simulink model "Autopilot"  (Simulink 8.0)
settings: configuration reference "configSetObj_autopilot" (kept outside this file)
undefined symbols (not defined in the file or in its folder): dispGain, intGain, rateGain
settings Model: Creator=The MathWorks Inc.  LastModifiedBy=klindqvi  CovMetricSettings=dcmtrwe  CovHTMLOptions=-aTS=1 -bRG=1 -bTC=1 -hTR=0 -nFC=0 -scm=1 -bcm=1 -xEv=0  CovSaveSingleToWorkspaceVar=off  CovCumulativeReport=on  CovModelRefEnable=off  ExtModeTrigMode=oneshot  ExtModeArmWhenConnect=off  ExtModeAutoUpdateStatusClock=off
settings ConfigSet: SourceLocation=Base Workspace

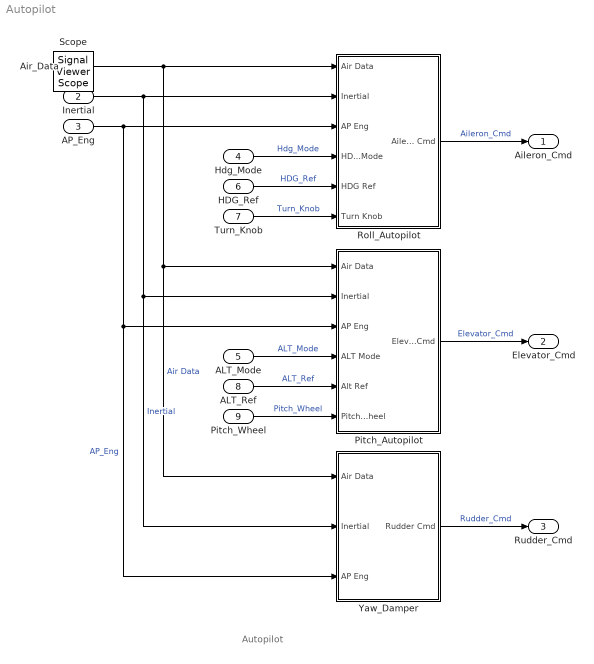
== system Autopilot ==
  note: Autopilot
  Air_Data : Inport  OutDataTypeStr=Bus: slBus_AirData  SampleTime=[0.025000000000000001,0]  BusOutputAsStruct=on
  Inertial : Inport  Port=2  OutDataTypeStr=Bus: slBus_Inertial  SampleTime=[0.025000000000000001,0]  BusOutputAsStruct=on
  AP_Eng : Inport  Port=3  OutDataTypeStr=boolean  PortDimensions=1  SampleTime=[0.025000000000000001,0]
  Hdg_Mode : Inport  Port=4  OutDataTypeStr=boolean  PortDimensions=1  SampleTime=[0.025000000000000001,0]
  ALT_Mode : Inport  Port=5  OutDataTypeStr=boolean  PortDimensions=1  SampleTime=[0.025000000000000001,0]
  HDG_Ref : Inport  Port=6  OutDataTypeStr=double  PortDimensions=1  SampleTime=[0.025000000000000001,0]
  Turn_Knob : Inport  Port=7  OutDataTypeStr=double  PortDimensions=1  SampleTime=[0.025000000000000001,0]
  ALT_Ref : Inport  Port=8  OutDataTypeStr=double  PortDimensions=1  SampleTime=[0.025000000000000001,0]
  Pitch_Wheel : Inport  Port=9  OutDataTypeStr=double  PortDimensions=1  SampleTime=[0.025000000000000001,0]
  Pitch_Autopilot : Subsystem  TreatAsAtomicUnit=on
  Roll_Autopilot : Subsystem  TreatAsAtomicUnit=on
  Yaw_Damper : Subsystem  TreatAsAtomicUnit=on
  Aileron_Cmd : Outport  OutDataTypeStr=double  PortDimensions=1  SampleTime=[0.025000000000000001,0]
  Elevator_Cmd : Outport  Port=2  OutDataTypeStr=double  PortDimensions=1  SampleTime=[0.025000000000000001,0]
  Rudder_Cmd : Outport  Port=3  OutDataTypeStr=double  PortDimensions=1  SampleTime=[0.025000000000000001,0]
  Scope : SignalViewerScope  IOType=viewer  RefreshTime=0.035000
  wires:
  AP_Eng/1 -> Yaw_Damper/3(AP Eng), Pitch_Autopilot/3(AP Eng), Roll_Autopilot/3(AP Eng)  "AP_Eng"
  Pitch_Wheel/1 -> Pitch_Autopilot/6(Pitch Wheel)  "Pitch_Wheel"
  ALT_Ref/1 -> Pitch_Autopilot/5(Alt Ref)  "ALT_Ref"
  ALT_Mode/1 -> Pitch_Autopilot/4(ALT Mode)  "ALT_Mode"
  Turn_Knob/1 -> Roll_Autopilot/6(Turn Knob)  "Turn_Knob"
  HDG_Ref/1 -> Roll_Autopilot/5(HDG Ref)  "HDG_Ref"
  Hdg_Mode/1 -> Roll_Autopilot/4(HDG Mode)  "Hdg_Mode"
  Inertial/1 -> Yaw_Damper/2(Inertial), Pitch_Autopilot/2(Inertial), Roll_Autopilot/2(Inertial)  "Inertial"
  Air_Data/1 -> Yaw_Damper/1(Air Data), Pitch_Autopilot/1(Air Data), Roll_Autopilot/1(Air Data)  "Air Data"
  Yaw_Damper/1(Rudder Cmd) -> Rudder_Cmd/1  "Rudder_Cmd"
  Pitch_Autopilot/1(Elevator_Cmd) -> Elevator_Cmd/1  "Elevator_Cmd"
  Roll_Autopilot/1(Aileron Cmd) -> Aileron_Cmd/1  "Aileron_Cmd"

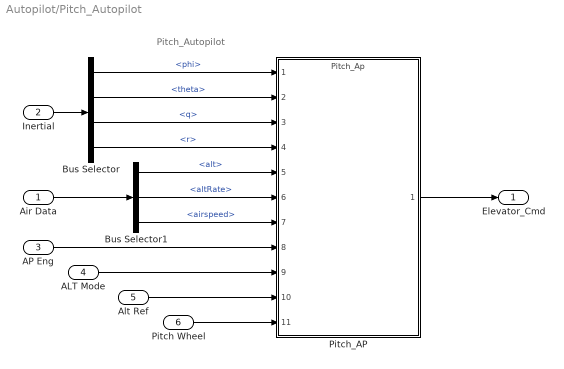
== system Autopilot/Pitch_Autopilot ==
  note: Pitch_Autopilot
  Air Data : Inport
  Inertial : Inport  Port=2
  AP Eng : Inport  Port=3
  ALT Mode : Inport  Port=4
  Alt Ref : Inport  Port=5
  Pitch Wheel : Inport  Port=6
  Bus Selector : BusSelector  OutputSignals=phi,theta,q,r
  Bus Selector1 : BusSelector  OutputSignals=alt,altRate,airspeed
  Pitch_AP : ModelReference  ModelNameDialog=Pitch_Ap  ParameterArgumentNames=dispGain,intGain,rateGain  ParameterArgumentValues=2.0, 0.5, 2.0  SimulationMode=Normal  ModelReferenceVersion=1.97  CopyOfModelName=Pitch_Ap  DefaultDataLogging=off
  Elevator_Cmd : Outport
  wires:
  Pitch Wheel/1 -> Pitch_AP/11
  Alt Ref/1 -> Pitch_AP/10
  ALT Mode/1 -> Pitch_AP/9
  AP Eng/1 -> Pitch_AP/8
  Bus Selector1/3 -> Pitch_AP/7  "<airspeed>"
  Bus Selector1/2 -> Pitch_AP/6  "<altRate>"
  Bus Selector1/1 -> Pitch_AP/5  "<alt>"
  Air Data/1 -> Bus Selector1/1
  Bus Selector/4 -> Pitch_AP/4  "<r>"
  Bus Selector/3 -> Pitch_AP/3  "<q>"
  Bus Selector/2 -> Pitch_AP/2  "<theta>"
  Bus Selector/1 -> Pitch_AP/1  "<phi>"
  Inertial/1 -> Bus Selector/1
  Pitch_AP/1 -> Elevator_Cmd/1

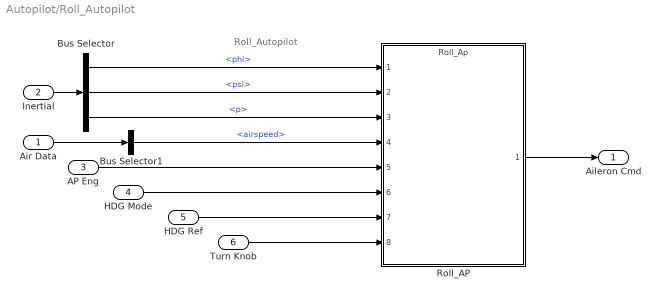
== system Autopilot/Roll_Autopilot ==
  note: Roll_Autopilot
  Air Data : Inport
  Inertial : Inport  Port=2
  AP Eng : Inport  Port=3
  HDG Mode : Inport  Port=4
  HDG Ref : Inport  Port=5
  Turn Knob : Inport  Port=6
  Bus Selector : BusSelector  OutputSignals=phi,psi,p
  Bus Selector1 : BusSelector  OutputSignals=airspeed
  Roll_AP : ModelReference  ModelNameDialog=Roll_Ap  SimulationMode=Normal  ModelReferenceVersion=1.244  CopyOfModelName=Roll_Ap  DefaultDataLogging=off
  Aileron Cmd : Outport
  wires:
  HDG Mode/1 -> Roll_AP/6
  AP Eng/1 -> Roll_AP/5
  HDG Ref/1 -> Roll_AP/7
  Turn Knob/1 -> Roll_AP/8
  Bus Selector1/1 -> Roll_AP/4  "<airspeed>"
  Air Data/1 -> Bus Selector1/1
  Bus Selector/3 -> Roll_AP/3  "<p>"
  Bus Selector/2 -> Roll_AP/2  "<psi>"
  Bus Selector/1 -> Roll_AP/1  "<phi>"
  Inertial/1 -> Bus Selector/1
  Roll_AP/1 -> Aileron Cmd/1

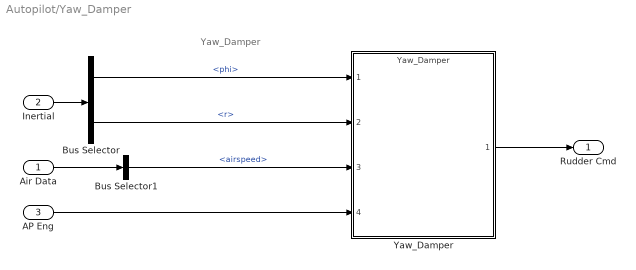
== system Autopilot/Yaw_Damper ==
  note: Yaw_Damper
  Air Data : Inport
  Inertial : Inport  Port=2
  AP Eng : Inport  Port=3
  Bus Selector : BusSelector  OutputSignals=phi,r
  Bus Selector1 : BusSelector  OutputSignals=airspeed
  Yaw_Damper : ModelReference  ModelNameDialog=Yaw_Damper  ParameterArgumentNames=rateGain  ParameterArgumentValues=1.0  SimulationMode=Normal  ModelReferenceVersion=1.71  CopyOfModelName=Yaw_Damper  DefaultDataLogging=off
  Rudder Cmd : Outport
  wires:
  AP Eng/1 -> Yaw_Damper/4
  Bus Selector/2 -> Yaw_Damper/2  "<r>"
  Bus Selector/1 -> Yaw_Damper/1  "<phi>"
  Inertial/1 -> Bus Selector/1
  Bus Selector1/1 -> Yaw_Damper/3  "<airspeed>"
  Air Data/1 -> Bus Selector1/1
  Yaw_Damper/1 -> Rudder Cmd/1
